simulink model "autopilot_fly"  (R2016a)
settings: Solver=VariableStepAuto  StartTime=0.0  StopTime=100  RelTol=1e-3
values from neighbouring files (symbols this model uses):
  U_trim = [-0.0594; 0.0005; -0.0010; 0.0978]    [run_autopilot.m]
  Va = 25    [run_autopilot.m]
  X_trim = [0; 0; -100.0000; 0.9993; -0.0011; 0.0332; 0.0186; 35.7388;             -0.0122; 2.3784; 0; 0; 0; -0.0300; 0; -0.0294; 0; 0.0978]    [run_autopilot.m]
libraries: X8_lib x2, simulink x2
settings Model: Creator=andreanv  LastModifiedBy=andreanv

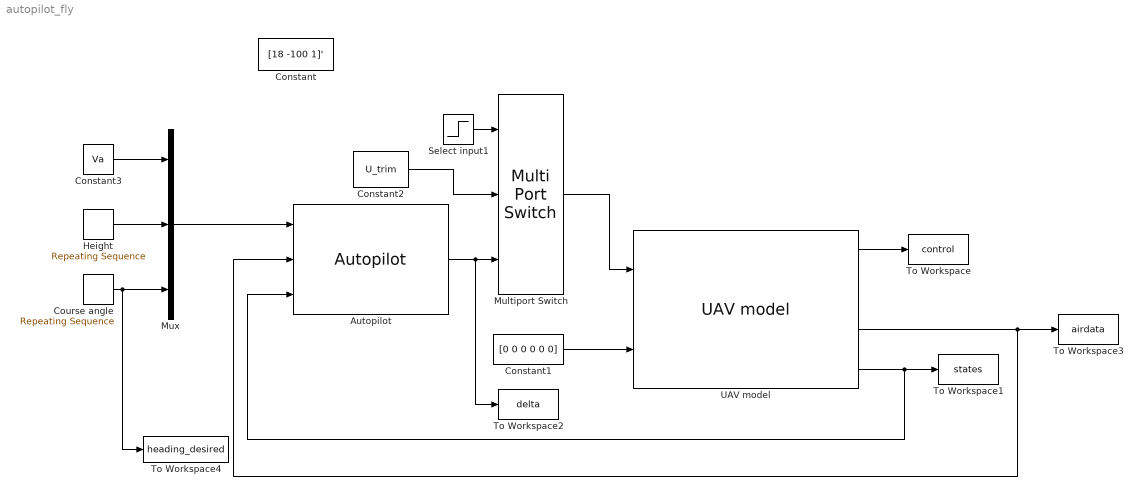
== system autopilot_fly ==
  Autopilot : X8_lib/Autopilot  param=param  X_trim=X_trim  U_trim=U_trim
  Constant : Constant  Value=[18 -100 1]'
  Constant1 : Constant  Value=[0 0 0 0 0 0]
  Constant2 : Constant  Value=U_trim
  Constant3 : Constant  Value=Va
  Course angle : simulink/Sources/Repeating Sequence  rep_seq_t=heading_time  rep_seq_y=heading_d
  Height : simulink/Sources/Repeating Sequence  rep_seq_t=[0 1]  rep_seq_y=[-100 -100]
  Multiport Switch : MultiPortSwitch  Inputs=2
  Mux : Mux  Inputs=3
  Select input1 : Step  Time=0  Before=1  After=2  SampleTime=0
  To Workspace : ToWorkspace  VariableName=control  SaveFormat=Timeseries  SampleTime=-1
  To Workspace1 : ToWorkspace  VariableName=states  SaveFormat=Timeseries  SampleTime=-1
  To Workspace2 : ToWorkspace  VariableName=delta  SaveFormat=Timeseries  SampleTime=-1
  To Workspace3 : ToWorkspace  VariableName=airdata  SaveFormat=Timeseries  SampleTime=-1
  To Workspace4 : ToWorkspace  VariableName=heading_desired  SaveFormat=Timeseries  SampleTime=-1
  UAV model : X8_lib/UAV model  param=param  pos0=X_trim(1:3)'  quat0=X_trim(4:7)'  vel0=X_trim(8:10)'  rate0=X_trim(11:13)'  servoR_pos0=X_trim(14)  servoR_vel0=X_trim(15)  servoL_pos0=X_trim(16)  servoL_vel0=X_trim(17)  motor_speed0=X_trim(18)
  wires:
  Constant1/1 -> UAV model/2
  UAV model/1 -> To Workspace/1
  UAV model/4 -> Autopilot/3, To Workspace1/1
  Constant2/1 -> Multiport Switch/2
  Select input1/1 -> Multiport Switch/1
  Multiport Switch/1 -> UAV model/1
  Autopilot/1 -> To Workspace2/1, Multiport Switch/3
  UAV model/3 -> Autopilot/2, To Workspace3/1
  Mux/1 -> Autopilot/1
  Course angle/1 -> Mux/3, To Workspace4/1
  Height/1 -> Mux/2
  Constant3/1 -> Mux/1
